simulink library "base_lib"  (R2023a)
settings: Solver=VariableStepAuto  StartTime=0.0  StopTime=10.0  RelTol=1e-3
(part 1 of 4)
settings Model: Creator=maxjo65  LastModifiedBy=maxjo65
settings SolverCC: AlgebraicLoopSolver=TrustRegion
settings OptimizationCC: ReuseModelBlockBuffer=off
settings DebuggingCC: UnconnectedInputMsg=warning  UnconnectedOutputMsg=warning  UnconnectedLineMsg=warning
settings ModelReferenceCC: EnableRefExpFcnMdlSchedulingChecks=on
settings RTWCC: DLArmComputeVersion=19.05

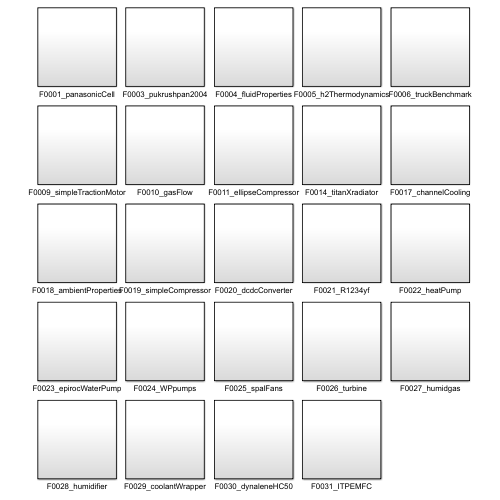
[thumbnail: Simulink's stored preview of the top-level diagram]
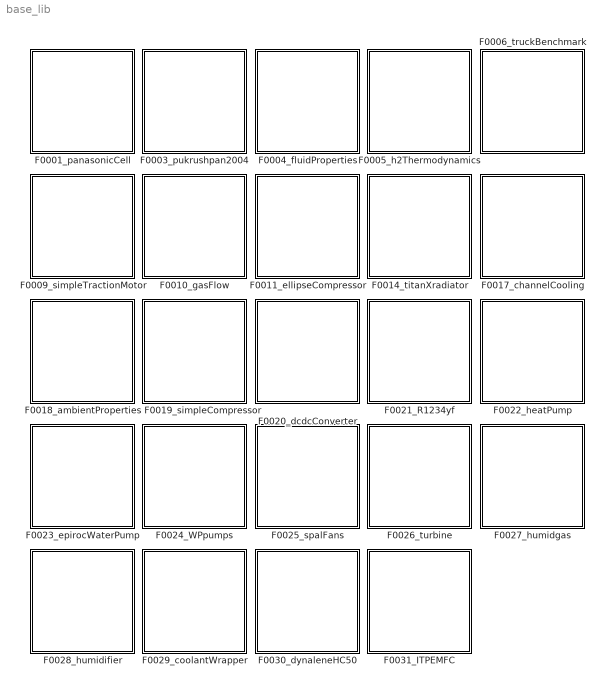
== system base_lib ==
  F0001_panasonicCell : Subsystem
  F0003_pukrushpan2004 : Subsystem
  F0004_fluidProperties : Subsystem
  F0005_h2Thermodynamics : Subsystem
  F0006_truckBenchmark : Subsystem
  F0009_simpleTractionMotor : Subsystem
  F0010_gasFlow : Subsystem
  F0011_ellipseCompressor : Subsystem
  F0014_titanXradiator : Subsystem
  F0017_channelCooling : Subsystem
  F0018_ambientProperties : Subsystem
  F0019_simpleCompressor : Subsystem
  F0020_dcdcConverter : Subsystem
  F0021_R1234yf : Subsystem
  F0022_heatPump : Subsystem
  F0023_epirocWaterPump : Subsystem
  F0024_WPpumps : Subsystem
  F0025_spalFans : Subsystem
  F0026_turbine : Subsystem
  F0027_humidgas : Subsystem
  F0028_humidifier : Subsystem
  F0029_coolantWrapper : Subsystem
  F0030_dynaleneHC50 : Subsystem
  F0031_ITPEMFC : Subsystem

== system base_lib/F0001_panasonicCell ==
  F0001_cellCapacity.m : MATLAB Function  TreatAsAtomicUnit=on
  F0001_dynamicVoltage.m : MATLAB Function  TreatAsAtomicUnit=on
  F0001_ocvSOC.m : MATLAB Function  TreatAsAtomicUnit=on

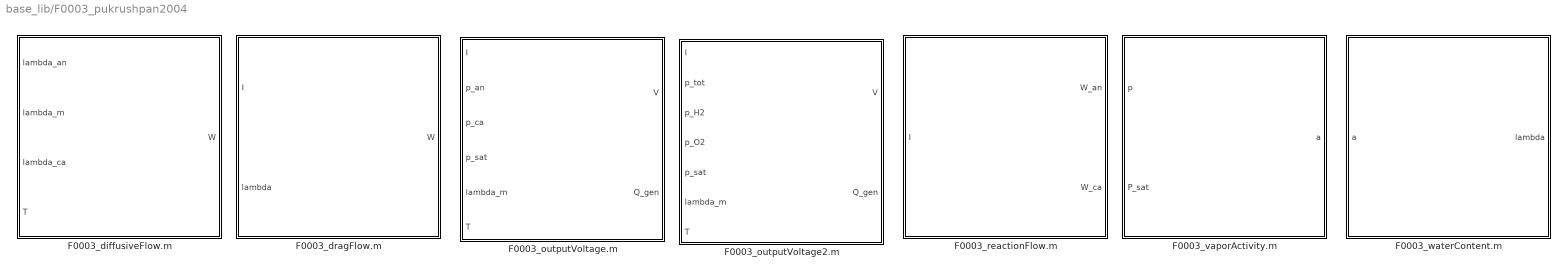
== system base_lib/F0003_pukrushpan2004 ==
  F0003_diffusiveFlow.m : MATLAB Function  TreatAsAtomicUnit=on
  F0003_dragFlow.m : MATLAB Function  TreatAsAtomicUnit=on
  F0003_outputVoltage.m : MATLAB Function  TreatAsAtomicUnit=on
  F0003_outputVoltage2.m : MATLAB Function  TreatAsAtomicUnit=on
  F0003_reactionFlow.m : MATLAB Function  TreatAsAtomicUnit=on
  F0003_vaporActivity.m : MATLAB Function  TreatAsAtomicUnit=on
  F0003_waterContent.m : MATLAB Function  TreatAsAtomicUnit=on

== system base_lib/F0004_fluidProperties ==
  F0004_mixtureMassSpecificHeat.m : MATLAB Function  TreatAsAtomicUnit=on
  F0004_pressureToMass.m : MATLAB Function  TreatAsAtomicUnit=on
  F0004_temperatureToEnthalpy.m : MATLAB Function  TreatAsAtomicUnit=on
  F0004_vaporSaturationConcentration.m : MATLAB Function  TreatAsAtomicUnit=on

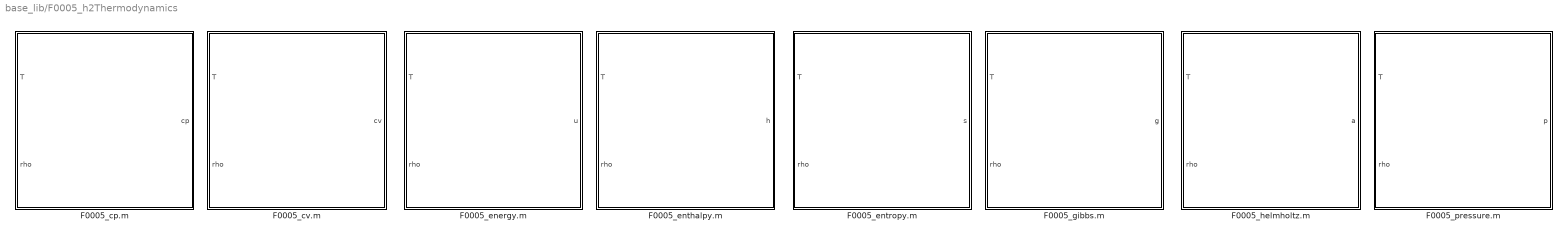
== system base_lib/F0005_h2Thermodynamics ==
  F0005_cp.m : MATLAB Function  TreatAsAtomicUnit=on
  F0005_cv.m : MATLAB Function  TreatAsAtomicUnit=on
  F0005_energy.m : MATLAB Function  TreatAsAtomicUnit=on
  F0005_enthalpy.m : MATLAB Function  TreatAsAtomicUnit=on
  F0005_entropy.m : MATLAB Function  TreatAsAtomicUnit=on
  F0005_gibbs.m : MATLAB Function  TreatAsAtomicUnit=on
  F0005_helmholtz.m : MATLAB Function  TreatAsAtomicUnit=on
  F0005_pressure.m : MATLAB Function  TreatAsAtomicUnit=on

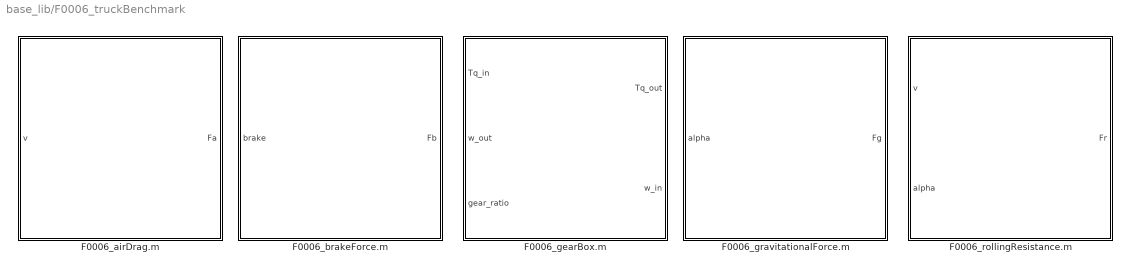
== system base_lib/F0006_truckBenchmark ==
  F0006_airDrag.m : MATLAB Function  TreatAsAtomicUnit=on
  F0006_brakeForce.m : MATLAB Function  TreatAsAtomicUnit=on
  F0006_gearBox.m : MATLAB Function  TreatAsAtomicUnit=on
  F0006_gravitationalForce.m : MATLAB Function  TreatAsAtomicUnit=on
  F0006_rollingResistance.m : MATLAB Function  TreatAsAtomicUnit=on

== system base_lib/F0009_simpleTractionMotor ==
  F0009_currentDemand.m : MATLAB Function  TreatAsAtomicUnit=on
  F0009_torque.m : MATLAB Function  TreatAsAtomicUnit=on
  F0009_torqueLimit.m : MATLAB Function  TreatAsAtomicUnit=on

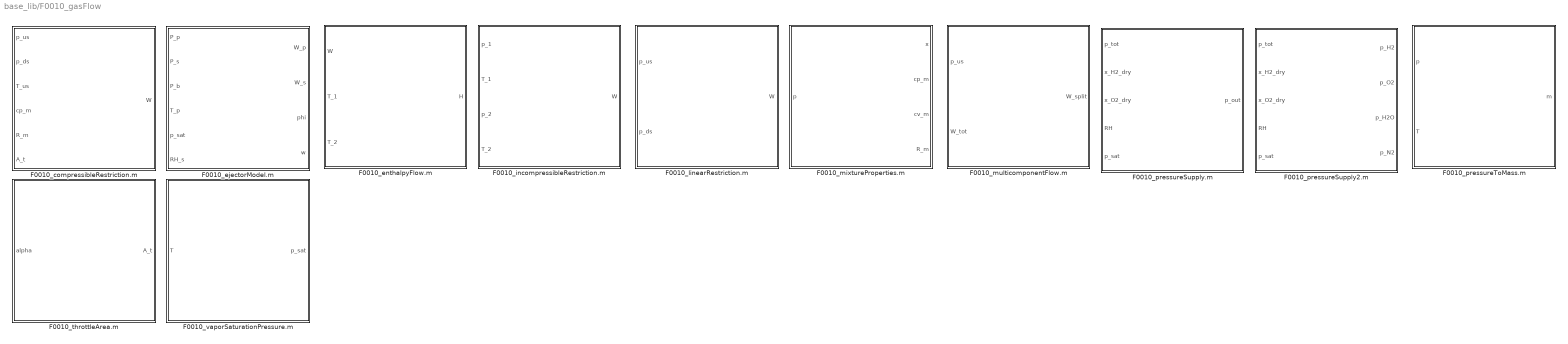
== system base_lib/F0010_gasFlow ==
  F0010_compressibleRestriction.m : MATLAB Function  TreatAsAtomicUnit=on
  F0010_ejectorModel.m : MATLAB Function  TreatAsAtomicUnit=on
  F0010_enthalpyFlow.m : MATLAB Function  TreatAsAtomicUnit=on
  F0010_incompressibleRestriction.m : MATLAB Function  TreatAsAtomicUnit=on
  F0010_linearRestriction.m : MATLAB Function  TreatAsAtomicUnit=on
  F0010_mixtureProperties.m : MATLAB Function  TreatAsAtomicUnit=on
  F0010_multicomponentFlow.m : MATLAB Function  TreatAsAtomicUnit=on
  F0010_pressureSupply.m : MATLAB Function  TreatAsAtomicUnit=on
  F0010_pressureSupply2.m : MATLAB Function  TreatAsAtomicUnit=on
  F0010_pressureToMass.m : MATLAB Function  TreatAsAtomicUnit=on
  F0010_throttleArea.m : MATLAB Function  TreatAsAtomicUnit=on
  F0010_vaporSaturationPressure.m : MATLAB Function  TreatAsAtomicUnit=on

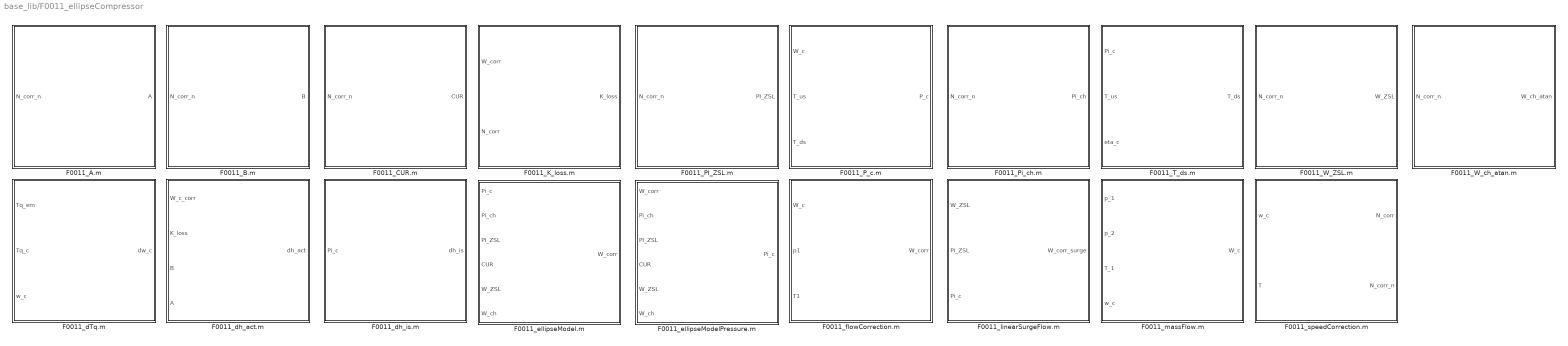
== system base_lib/F0011_ellipseCompressor ==
  F0011_A.m : MATLAB Function  TreatAsAtomicUnit=on
  F0011_B.m : MATLAB Function  TreatAsAtomicUnit=on
  F0011_CUR.m : MATLAB Function  TreatAsAtomicUnit=on
  F0011_K_loss.m : MATLAB Function  TreatAsAtomicUnit=on
  F0011_PI_ZSL.m : MATLAB Function  TreatAsAtomicUnit=on
  F0011_P_c.m : MATLAB Function  TreatAsAtomicUnit=on
  F0011_Pi_ch.m : MATLAB Function  TreatAsAtomicUnit=on
  F0011_T_ds.m : MATLAB Function  TreatAsAtomicUnit=on
  F0011_W_ZSL.m : MATLAB Function  TreatAsAtomicUnit=on
  F0011_W_ch_atan.m : MATLAB Function  TreatAsAtomicUnit=on
  F0011_dTq.m : MATLAB Function  TreatAsAtomicUnit=on
  F0011_dh_act.m : MATLAB Function  TreatAsAtomicUnit=on
  F0011_dh_is.m : MATLAB Function  TreatAsAtomicUnit=on
  F0011_ellipseModel.m : MATLAB Function  TreatAsAtomicUnit=on
  F0011_ellipseModelPressure.m : MATLAB Function  TreatAsAtomicUnit=on
  F0011_flowCorrection.m : MATLAB Function  TreatAsAtomicUnit=on
  F0011_linearSurgeFlow.m : MATLAB Function  TreatAsAtomicUnit=on
  F0011_massFlow.m : MATLAB Function  TreatAsAtomicUnit=on
  F0011_speedCorrection.m : MATLAB Function  TreatAsAtomicUnit=on

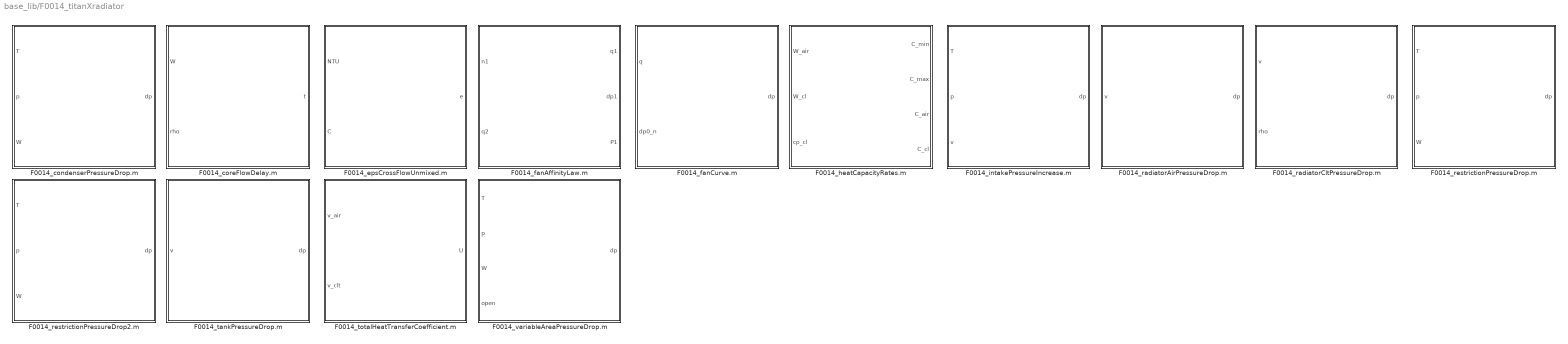
== system base_lib/F0014_titanXradiator ==
  F0014_condenserPressureDrop.m : MATLAB Function  TreatAsAtomicUnit=on
  F0014_coreFlowDelay.m : MATLAB Function  TreatAsAtomicUnit=on
  F0014_epsCrossFlowUnmixed.m : MATLAB Function  TreatAsAtomicUnit=on
  F0014_fanAffinityLaw.m : MATLAB Function  TreatAsAtomicUnit=on
  F0014_fanCurve.m : MATLAB Function  TreatAsAtomicUnit=on
  F0014_heatCapacityRates.m : MATLAB Function  TreatAsAtomicUnit=on
  F0014_intakePressureIncrease.m : MATLAB Function  TreatAsAtomicUnit=on
  F0014_radiatorAirPressureDrop.m : MATLAB Function  TreatAsAtomicUnit=on
  F0014_radiatorCltPressureDrop.m : MATLAB Function  TreatAsAtomicUnit=on
  F0014_restrictionPressureDrop.m : MATLAB Function  TreatAsAtomicUnit=on
  F0014_restrictionPressureDrop2.m : MATLAB Function  TreatAsAtomicUnit=on
  F0014_tankPressureDrop.m : MATLAB Function  TreatAsAtomicUnit=on
  F0014_totalHeatTransferCoefficient.m : MATLAB Function  TreatAsAtomicUnit=on
  F0014_variableAreaPressureDrop.m : MATLAB Function  TreatAsAtomicUnit=on

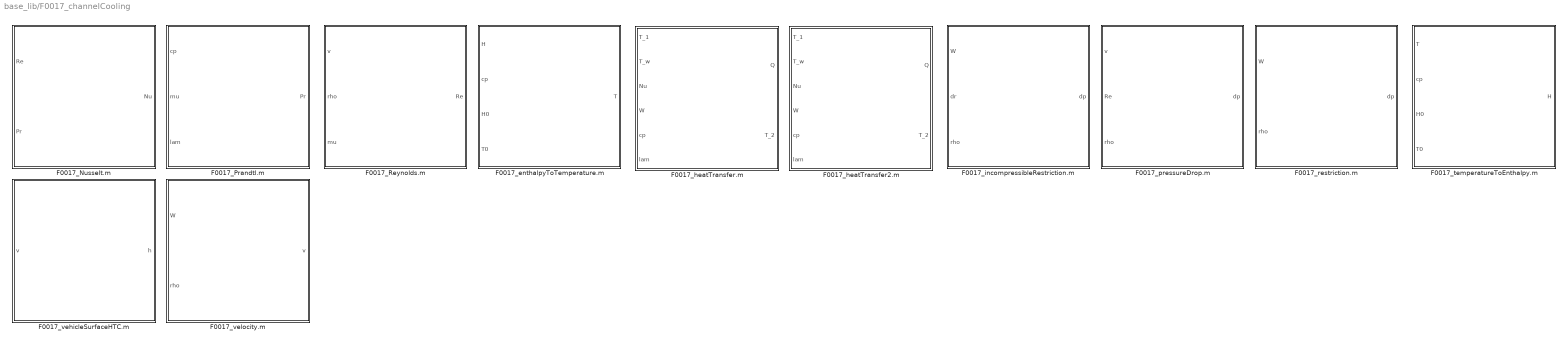
== system base_lib/F0017_channelCooling ==
  F0017_Nusselt.m : MATLAB Function  TreatAsAtomicUnit=on
  F0017_Prandtl.m : MATLAB Function  TreatAsAtomicUnit=on
  F0017_Reynolds.m : MATLAB Function  TreatAsAtomicUnit=on
  F0017_enthalpyToTemperature.m : MATLAB Function  TreatAsAtomicUnit=on
  F0017_heatTransfer.m : MATLAB Function  TreatAsAtomicUnit=on
  F0017_heatTransfer2.m : MATLAB Function  TreatAsAtomicUnit=on
  F0017_incompressibleRestriction.m : MATLAB Function  TreatAsAtomicUnit=on
  F0017_pressureDrop.m : MATLAB Function  TreatAsAtomicUnit=on
  F0017_restriction.m : MATLAB Function  TreatAsAtomicUnit=on
  F0017_temperatureToEnthalpy.m : MATLAB Function  TreatAsAtomicUnit=on
  F0017_vehicleSurfaceHTC.m : MATLAB Function  TreatAsAtomicUnit=on
  F0017_velocity.m : MATLAB Function  TreatAsAtomicUnit=on

== system base_lib/F0018_ambientProperties ==
  F0018_troposphereModel.m : MATLAB Function  TreatAsAtomicUnit=on

== system base_lib/F0019_simpleCompressor ==
  F0007_compressorPower.m : MATLAB Function  TreatAsAtomicUnit=on
  F0007_compressorTemperature.m : MATLAB Function  TreatAsAtomicUnit=on

== system base_lib/F0020_dcdcConverter ==
  F0020_dcdcConverter.m : MATLAB Function  TreatAsAtomicUnit=on

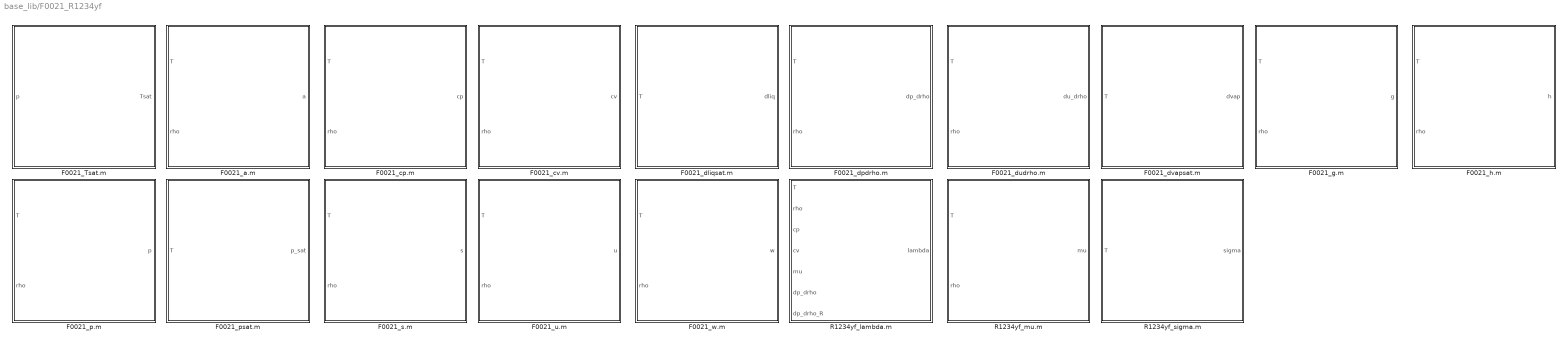
== system base_lib/F0021_R1234yf ==
  F0021_Tsat.m : MATLAB Function  TreatAsAtomicUnit=on
  F0021_a.m : MATLAB Function  TreatAsAtomicUnit=on
  F0021_cp.m : MATLAB Function  TreatAsAtomicUnit=on
  F0021_cv.m : MATLAB Function  TreatAsAtomicUnit=on
  F0021_dliqsat.m : MATLAB Function  TreatAsAtomicUnit=on
  F0021_dpdrho.m : MATLAB Function  TreatAsAtomicUnit=on
  F0021_dudrho.m : MATLAB Function  TreatAsAtomicUnit=on
  F0021_dvapsat.m : MATLAB Function  TreatAsAtomicUnit=on
  F0021_g.m : MATLAB Function  TreatAsAtomicUnit=on
  F0021_h.m : MATLAB Function  TreatAsAtomicUnit=on
  F0021_p.m : MATLAB Function  TreatAsAtomicUnit=on
  F0021_psat.m : MATLAB Function  TreatAsAtomicUnit=on
  F0021_s.m : MATLAB Function  TreatAsAtomicUnit=on
  F0021_u.m : MATLAB Function  TreatAsAtomicUnit=on
  F0021_w.m : MATLAB Function  TreatAsAtomicUnit=on
  R1234yf_lambda.m : MATLAB Function  TreatAsAtomicUnit=on
  R1234yf_mu.m : MATLAB Function  TreatAsAtomicUnit=on
  R1234yf_sigma.m : MATLAB Function  TreatAsAtomicUnit=on

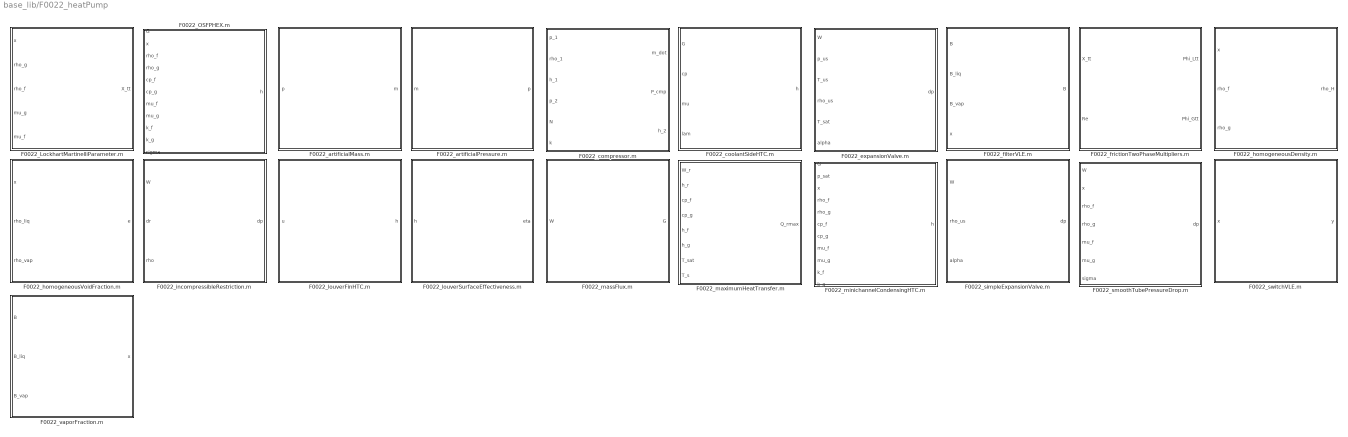
== system base_lib/F0022_heatPump ==
  F0022_LockhartMartinelliParameter.m : MATLAB Function  TreatAsAtomicUnit=on
  F0022_OSFPHEX.m : MATLAB Function  TreatAsAtomicUnit=on
  F0022_artificialMass.m : MATLAB Function  TreatAsAtomicUnit=on
  F0022_artificialPressure.m : MATLAB Function  TreatAsAtomicUnit=on
  F0022_compressor.m : MATLAB Function  TreatAsAtomicUnit=on
  F0022_coolantSideHTC.m : MATLAB Function  TreatAsAtomicUnit=on
  F0022_expansionValve.m : MATLAB Function  TreatAsAtomicUnit=on
  F0022_filterVLE.m : MATLAB Function  TreatAsAtomicUnit=on
  F0022_frictionTwoPhaseMultipliers.m : MATLAB Function  TreatAsAtomicUnit=on
  F0022_homogeneousDensity.m : MATLAB Function  TreatAsAtomicUnit=on
  F0022_homogeneousVoidFraction.m : MATLAB Function  TreatAsAtomicUnit=on
  F0022_incompressibleRestriction.m : MATLAB Function  TreatAsAtomicUnit=on
  F0022_louverFinHTC.m : MATLAB Function  TreatAsAtomicUnit=on
  F0022_louverSurfaceEffectiveness.m : MATLAB Function  TreatAsAtomicUnit=on
  F0022_massFlux.m : MATLAB Function  TreatAsAtomicUnit=on
  F0022_maximumHeatTransfer.m : MATLAB Function  TreatAsAtomicUnit=on
  F0022_minichannelCondensingHTC.m : MATLAB Function  TreatAsAtomicUnit=on
  F0022_simpleExpansionValve.m : MATLAB Function  TreatAsAtomicUnit=on
  F0022_smoothTubePressureDrop.m : MATLAB Function  TreatAsAtomicUnit=on
  F0022_switchVLE.m : MATLAB Function  TreatAsAtomicUnit=on
  F0022_vaporFraction.m : MATLAB Function  TreatAsAtomicUnit=on

== system base_lib/F0023_epirocWaterPump ==
  F0023_current.m : MATLAB Function  TreatAsAtomicUnit=on
  F0023_pressure.m : MATLAB Function  TreatAsAtomicUnit=on
  F0023_speed.m : MATLAB Function  TreatAsAtomicUnit=on

== system base_lib/F0024_WPpumps ==
  F0024_powerWP120.m : MATLAB Function  TreatAsAtomicUnit=on
  F0024_powerWP150.m : MATLAB Function  TreatAsAtomicUnit=on
  F0024_pressureWP120.m : MATLAB Function  TreatAsAtomicUnit=on
  F0024_pressureWP150.m : MATLAB Function  TreatAsAtomicUnit=on

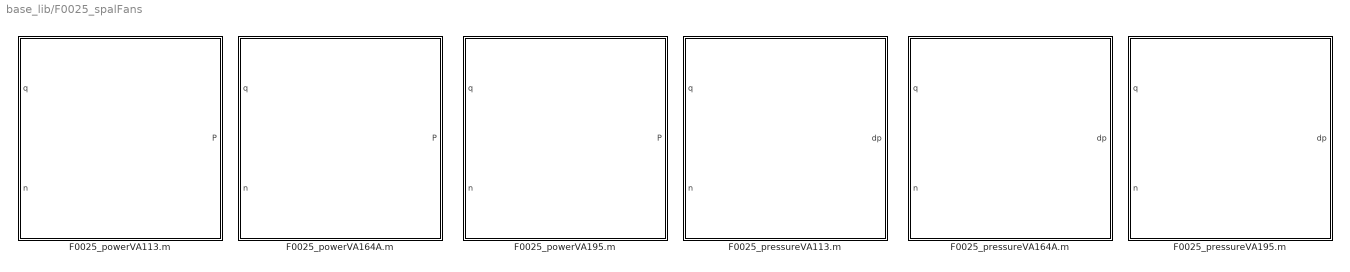
== system base_lib/F0025_spalFans ==
  F0025_powerVA113.m : MATLAB Function  TreatAsAtomicUnit=on
  F0025_powerVA164A.m : MATLAB Function  TreatAsAtomicUnit=on
  F0025_powerVA195.m : MATLAB Function  TreatAsAtomicUnit=on
  F0025_pressureVA113.m : MATLAB Function  TreatAsAtomicUnit=on
  F0025_pressureVA164A.m : MATLAB Function  TreatAsAtomicUnit=on
  F0025_pressureVA195.m : MATLAB Function  TreatAsAtomicUnit=on

== system base_lib/F0026_turbine ==
  F0026_turbine.m : MATLAB Function  TreatAsAtomicUnit=on

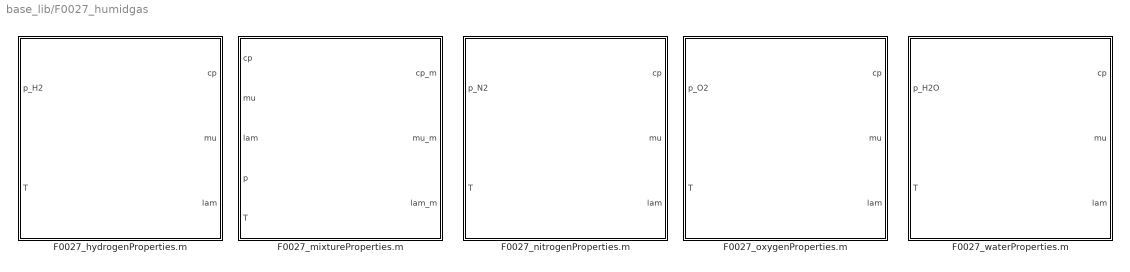
== system base_lib/F0027_humidgas ==
  F0027_hydrogenProperties.m : MATLAB Function  TreatAsAtomicUnit=on
  F0027_mixtureProperties.m : MATLAB Function  TreatAsAtomicUnit=on
  F0027_nitrogenProperties.m : MATLAB Function  TreatAsAtomicUnit=on
  F0027_oxygenProperties.m : MATLAB Function  TreatAsAtomicUnit=on
  F0027_waterProperties.m : MATLAB Function  TreatAsAtomicUnit=on

== system base_lib/F0028_humidifier ==
  F0028_absHumidity.m : MATLAB Function  TreatAsAtomicUnit=on
  F0028_heatTransfer.m : MATLAB Function  TreatAsAtomicUnit=on
  F0028_massTransfer.m : MATLAB Function  TreatAsAtomicUnit=on
  F0028_minWcp.m : MATLAB Function  TreatAsAtomicUnit=on

== system base_lib/F0029_coolantWrapper ==
  F0029_density.m : MATLAB Function  TreatAsAtomicUnit=on
  F0029_heatCapacity.m : MATLAB Function  TreatAsAtomicUnit=on
  F0029_thermalConductivity.m : MATLAB Function  TreatAsAtomicUnit=on
  F0029_viscosity.m : MATLAB Function  TreatAsAtomicUnit=on

== system base_lib/F0030_dynaleneHC50 ==
  F0030_density.m : MATLAB Function  TreatAsAtomicUnit=on
  F0030_heatCapacity.m : MATLAB Function  TreatAsAtomicUnit=on
  F0030_thermalConductivity.m : MATLAB Function  TreatAsAtomicUnit=on
  F0030_viscosity.m : MATLAB Function  TreatAsAtomicUnit=on

== system base_lib/F0031_ITPEMFC ==
  F0031_ITPEMFC.m : MATLAB Function  TreatAsAtomicUnit=on

== matlab function base_lib/F0022_heatPump/F0022_filterVLE.m ==
  data: B input; B output; B_liq input; B_vap input; x input
function B = F0022_filterVLE(B, B_liq, B_vap, x)

% assign saturated property
B( x > 0 & x < 1) = x .* B_vap + (1-x) .* B_liq;


end

== matlab function base_lib/F0022_heatPump/F0022_frictionTwoPhaseMultipliers.m ==
  data: X_tt input; Phi_Ltt output; Re input; Phi_Gtt output
function [Phi_Ltt, Phi_Gtt] = F0022_frictionTwoPhaseMultipliers(X_tt, Re)


% Liquid
Phi_Ltt = 1 + C./X_tt + 1./X_tt.^2;

% Gas
Phi_Gtt = 1 + C.*X_tt + X_tt.^2;



end

== matlab function base_lib/F0022_heatPump/F0022_homogeneousDensity.m ==
  data: x input; rho_H output; rho_f input; rho_g input
function rho_H = F0022_homogeneousDensity(x, rho_f, rho_g)

% thermopedia.com /cn/content/37/
rho_h = rho_f .* rho_g ./ ( x.* rho_f + (1-x) .* rho_g );

end

== matlab function base_lib/F0022_heatPump/F0022_homogeneousVoidFraction.m ==
  data: x input; e output; rho_liq input; rho_vap input
function e = F0022_homogeneousVoidFraction(x, rho_liq, rho_vap)

% from Engineering Data Book II, Wolverine Tube Inc.

e = 1 ./ ( 1 + (1-x)./x .* rho_vap ./ rho_liq );


end

== matlab function base_lib/F0022_heatPump/F0022_incompressibleRestriction.m ==
  data: W input; dp output; dr input; rho input; par parameter
function dp = F0022_incompressibleRestriction(W, dr, rho, par)

% parameters
C_d = par.C_d;
d   = par.d;

% restriction area
Ar = dr.^2 * pi / 4;

% diameter ratio
beta = dr./d;

% volumetric flow
Q = W ./ rho;

% pressure drop
dp = 1/2 .* rho .* (1 - beta.^4) .* (Q ./ (C_d .* Ar)).^2;

== matlab function base_lib/F0021_R1234yf/F0021_w.m ==
  data: T input; w output; rho input
function w = F0021_w(T,rho)
%R1234yf_w
%    W = R1234yf_w(T,RHO)

%    This function was generated by the Symbolic Math Toolbox version 9.3.
%    16-Oct-2023 15:47:53

t2 = T.^2;
t3 = rho.^2;
t4 = rho.^3;
t6 = rho.^5;
t8 = rho.^7;
t9 = 1.0./T;
t12 = rho./4.17e+3;
t17 = rho.*7.769784172661871e-3;
t25 = rho.*4.892086330935252e-4;
t30 = rho.*2.800959232613909e-3;
t32 = rho.*6.407673860911271e-4;
t33 = rho.*5.059952038369305e-4;
t5 = t3.^2;
t7 = t3.^3;
t10 = 1.0./t2;
t11 = t9.^3;
t13 = t9.*7.18e+2;
t14 = t9.*8.77e+2;
t15 = t9.*1.755e+3;
t16 = t9.*4.465e+3;
t18 = -t12;
t23 = t9.*5.8856e+4;
t31 = t9.*3.6785e+2;
t34 = t9.*7.94556e+4;
t35 = t3./1.73889e+7;
t40 = t9.*1.044694e+3;
t41 = t12-4.1e+1./2.5e+1;
t49 = t9.*6.54773e+2;
t50 = t9.*1.699467e+3;
t51 = t12-9.1e+1./1.0e+2;
t52 = t12-8.9e+1./1.25e+2;
t53 = t12-3.59e+2./5.0e+2;
t68 = t12-6.77e+2./1.0e+3;
t69 = t17-5.3136e+1;
t78 = t25-1.45248;
t87 = t30-8.38624;
t92 = t32-2.43152;
t100 = t33-1.42847;
t123 = t4.*t9.*9.319180196722149e-10;
t19 = -t13;
t20 = -t14;
t21 = -t15;
t22 = -t16;
t24 = exp(t18);
t42 = -t35;
t43 = t31.^(3.0./2.0);
t44 = t31.^(2.0./5.0);
t45 = t31.^(5.0./2.0);
t46 = t31.^(7.0./2.0);
t47 = t31.^(7.0./5.0);
t54 = t31-6.0./5.0;
t55 = t31.^(1.0./2.0e+1);
t56 = t41.^2;
t57 = t31.^(8.0./2.5e+1);
t59 = t31.^(1.9e+1./2.5e+1);
t61 = t31.^(3.6e+1./2.5e+1);
t62 = t31.^(1.9e+1./5.0e+1);
t63 = t31.^(4.4e+1./2.5e+1);
t65 = t31.^(6.1e+1./2.5e+1);
t66 = t31.^(4.7e+1./5.0e+1);
t67 = t23-2.048e+2;
t70 = t31-3.2e+1./2.5e+1;
t71 = t31-2.3e+1./5.0e+1;
t72 = 1.0./t31.^(3.0./1.0e+2);
t73 = t51.^2;
t74 = t52.^2;
t75 = t53.^2;
t77 = t31.^(9.7e+1./1.0e+2);
t79 = t31-6.7e+1./1.0e+2;
t80 = t31-1.13e+2./1.0e+2;
t81 = t34-2.592e+2;
t82 = t68.^2;
t85 = t31.^(9.29e+2./1.0e+3);
t97 = t40-3.2092;
t103 = t49-8.188e-1;
t106 = t50-3.0954;
t26 = exp(t19);
t27 = exp(t20);
t28 = exp(t21);
t29 = exp(t22);
t48 = exp(t42);
t58 = t55.^21;
t60 = t57.^4;
t64 = t59.^3;
t76 = t54.^2;
t83 = t70.^2;
t84 = t71.^2;
t88 = t79.^2;
t89 = t80.^2;
t90 = t56.*(8.1e+1./5.0);
t95 = t74.*(5.1e+1./5.0e+1);
t99 = t75.*(1.46e+2./2.5e+1);
t101 = t73.*(1.67e+2./1.25e+2);
t107 = t82.*(2.11e+2./2.0e+2);
t115 = t57.*1.546958;
t119 = t85.*2.355237;
t120 = rho.*t66.*2.315508393285372e-4;
t130 = t3.*t62.*3.033007263254145e-8;
t133 = rho.*t24.*t77.*3.263914628297362e-4;
t136 = t3.*t24.*t77.*3.913566700596357e-8;
t36 = t26-1.0;
t37 = t27-1.0;
t38 = t28-1.0;
t39 = t29-1.0;
t86 = t76.*1.08e+2;
t93 = -t90;
t94 = t83.*8.0e+1;
t98 = -t95;
t102 = -t99;
t104 = -t101;
t105 = t84.*(8.9e+1./1.0e+2);
t109 = t89.*(7.1e+1./5.0e+1);
t110 = -t107;
t112 = t88.*(2.31e+2./1.0e+2);
t121 = -t119;
t122 = -t120;
t131 = t48.*t64.*1.210006;
t134 = rho.*t48.*t65.*3.342232613908873e-4;
t137 = t3.*t48.*t64.*1.391699302428561e-7;
t138 = -t136;
t139 = t3.*t48.*t63.*1.06569432224005e-7;
t141 = t4.*t48.*t65.*1.922049476337705e-11;
t142 = t5.*t48.*t63.*4.085726420264459e-15;
t143 = t7.*t24.*t58.*3.588938332192827e-23;
t145 = t8.*t24.*t58.*1.229509534838242e-27;
t91 = -t86;
t96 = -t94;
t108 = -t105;
t111 = -t109;
t113 = -t112;
t132 = -t131;
t135 = -t134;
t140 = -t139;
t144 = -t143;
t114 = t91+t93;
t117 = t96+t102;
t124 = t98+t111;
t126 = t104+t113;
t127 = t108+t110;
t116 = exp(t114);
t118 = exp(t117);
t125 = exp(t124);
t128 = exp(t126);
t129 = exp(t127);
t146 = t3.*t9.*t118.*7.283294189396684e-5;
t148 = rho.*t46.*t116.*1.644384172661871e-7;
t149 = t47.*t125.*1.389966;
t150 = t11.*t128.*2.377824987227386e+7;
t152 = t3.*t46.*t129.*3.407663509480186e-8;
t154 = t4.*t9.*t87.*t118.*5.821977769301905e-9;
t155 = t3.*t46.*t69.*t116.*1.971683660266032e-11;
t157 = rho.*t47.*t78.*t125.*3.333251798561151e-4;
t159 = rho.*t11.*t92.*t128.*5.702218194789895e+3;
t160 = t4.*t46.*t100.*t129.*2.723951646267135e-12;
t147 = -t146;
t151 = -t150;
t153 = -t152;
t156 = -t155;
t158 = -t157;
t161 = t115+t121+t122+t123+t130+t132+t133+t135+t137+t138+t140+t141+t142+t144+t145+t147+t148+t149+t151+t153+t154+t156+t158+t159+t160;
et1 = t66.*9.65567e-1+t138+t145-rho.*t62.*2.529528057553957e-4-t3.*t9.*1.165829442609941e-5-t24.*t77.*1.3610524;
et2 = t48.*t65.*1.393711-t46.*t116.*6.857082e-4+t87.*t154+t92.*t159+t100.*t160+rho.*t24.*t77.*6.527829256594724e-4+rho.*t48.*t63.*8.887890647482015e-4;
et3 = rho.*t48.*t64.*(-1.741015827338129e-3)+rho.*t9.*t118.*6.074267353956834e-1-rho.*t11.*t128.*1.52363270164786e+4+rho.*t47.*t125.*6.799833669064748e-4;
et4 = rho.*t46.*t129.*2.841991366906475e-4+t6.*t24.*t58.*8.979523707146454e-19-t7.*t24.*t58.*7.177876664385654e-23;
et5 = t4.*t48.*t63.*(-1.192623542075196e-10)-t3.*t48.*t65.*4.007473158164116e-7+t4.*t48.*t64.*6.674816798218516e-11+t6.*t48.*t63.*1.95958101691341e-18;
et6 = t5.*t48.*t65.*9.218462716247988e-15-t4.*t9.*t118.*6.800070034544626e-8+t3.*t46.*t116.*6.388255059261943e-10;
et7 = t4.*t46.*t129.*(-5.747537973623655e-12)-t11.*t92.*t128.*4.755649974454772e+7+t47.*t78.*t125.*2.779932+rho.*t46.*t69.*t116.*3.288768345323741e-7;
et8 = t3.*t9.*t87.*t118.*(-1.456658837879337e-4)-t3.*t46.*t100.*t129.*6.815327018960372e-8-rho.*t47.*t78.^2.*t125.*3.333251798561151e-4-t3.*t46.*t69.^2.*t116.*1.971683660266032e-11;
et9 = t4.*2.533418566459739e-12-t48.*t60.*2.75881368-t3.*t118.*1.979963079895795e-7-t10.*t128.*1.93923473200548e+5;
et10 = t44.*t125.*1.9459524+t67.*t146+t81.*t155+t97.*t157+t103.*t152+t106.*t150-rho.*t72.^2.*2.176577889688249e-4+t3.*1.0./t31.^(3.1e+1./5.0e+1).*1.152542760036575e-8+1.0./t31.^(1.7e+1./2.5e+1).*4.9502656e-1;
et11 = 1.0./t31.^(7.1e+1./1.0e+3).*(-2.188015173)+rho.*t24.*t72.*3.165997189448441e-4-rho.*t48.*t61.*8.155047577937649e-4+rho.*t45.*t116.*5.755344604316547e-7;
et12 = t7.*t24.*t55.*(-3.768385248802469e-23)+t8.*t24.*t55.*1.290985011580154e-27-t3.*t24.*t72.*3.796159699578467e-8;
et13 = t3.*t48.*t59.*(-1.875622007142488e-7)+t3.*t48.*t60.*3.173074409537118e-7+t5.*t48.*t59.*7.190878499665448e-15+t4.*t48.*t61.*4.689800722264001e-11;
et14 = t3.*t45.*t129.*(-1.192682228318065e-7)+t4.*t87.*t118.*1.582704300476255e-11-t47.*t97.*t125.*1.389966+rho.*t10.*t92.*t128.*4.650443002411223e+1;
et15 = rho.*t46.*t81.*t116.*(-1.644384172661871e-7)-rho.*t44.*t78.*t125.*4.666552517985612e-4-t3.*t45.*t69.*t116.*6.900892810931111e-11+t4.*t45.*t100.*t129.*9.533830761934972e-12;
et16 = rho.*t11.*t92.*t106.*t128.*(-5.702218194789895e+3)-t4.*t9.*t67.*t87.*t118.*5.821977769301905e-9-t4.*t46.*t100.*t103.*t129.*2.723951646267135e-12;
et17 = t2.*3.653734124219459e-5+1.0./t36.^2.*exp(t9.*-1.436e+3).*2.876052391546904e+1+1.0./t37.^2.*exp(t9.*-1.754e+3).*8.736380352244283+1.0./t38.^2.*exp(t9.*-3.51e+3).*1.696916093943165e+2+1.0./t39.^2.*exp(t9.*-8.93e+3).*2.990869359808914e+2+rho.*t72.^56.*8.072375558752998e-5;
et18 = rho.*1.0./t31.^1.071.*(-3.72539753676259e-5)-(t26.*2.876052391546904e+1)./t36-(t27.*8.736380352244283)./t37-(t28.*1.696916093943165e+2)./t38-(t29.*2.990869359808914e+2)./t39;
et19 = t4.*t72.^54.*5.712042455816759e-13-t3.*1.0./t31.^(5.3e+1./5.0e+1).*1.565883373876438e-9+rho.*t31.^(7.0./2.5e+1).*t48.*8.468300984172661e-4;
et20 = rho.*1.0./t55.^12.*t125.*(-1.866621007194245e-4)+t8.*t24.*1.0./t55.^19.*6.454925057900768e-29+t3.*t31.^(1.1e+1./2.5e+1).*t48.*1.408065768852544e-7;
et21 = t4.*t48.*t72.^8.*1.139466607056987e-11+t3.*t24.*1.0./t31.^(1.03e+2./1.0e+2).*1.13884790987354e-9+rho.*t9.*t128.*2.528445291510791e-1;
et22 = rho.*t11.*t128.*(-2.634424805992931e+4)+rho.*t47.*t125.*9.466435107913669e-4-t4.*t9.*t118.*9.315164430883049e-7;
et23 = t3.*t43.*t116.*(-1.725223202732778e-10)+t3.*t46.*t116.*4.258836706174629e-9+t4.*t43.*t129.*2.383457690483743e-11-t4.*t46.*t129.*4.8486339303555e-12;
et24 = t4.*t67.*t118.*(-3.165408600952511e-11)-rho.*t10.*t106.*t128.*9.300886004822446e+1+rho.*t44.*t97.*t125.*9.333105035971223e-4+t3.*t45.*t81.*t116.*1.380178562186222e-10;
et25 = t4.*t45.*t103.*t129.*(-1.906766152386994e-11)+rho.*t11.*t106.^2.*t128.*5.702218194789895e+3-rho.*t47.*t97.^2.*t125.*3.333251798561151e-4;
et26 = t4.*t9.*t67.^2.*t118.*5.821977769301905e-9-t3.*t46.*t81.^2.*t116.*1.971683660266032e-11+t4.*t46.*t103.^2.*t129.*2.723951646267135e-12;
w = sqrt(T.*((rho.*t161)./2.085e+3-(t3.*(et1+et2+et3+et4+et5+et6+et7+et8))./1.73889e+7+(t2.*(t12.*t161-rho.*t9.*(et9+et10+et11+et12+et13+et14+et15+et16).*8.821342925659472e-2+1.0).^2.*7.39023892439211e-6)./(et17+et18+et19+et20+et21+et22+et23+et24+et25+et26)+1.0).*7.290736472421491e+1);
end

== matlab function base_lib/F0004_fluidProperties/F0004_mixtureMassSpecificHeat.m ==
  data: p input; cp output; cv output; par parameter
function [cp, cv] = F0004_mixtureMassSpecificHeat(p, par)
% total pressure
p_tot = sum(p);

% mass specific heat capacity
cp_r  = par.cp_r;
cp_v  = par.cp_H2O;
cp_N2 = par.cp_N2;
R_r    = par.R_r;
R_H2O  = par.R_H2O;
R_N2   = par.R_N2;

% partial pressures
p_r  = p(1);
p_v  = p(2);
p_N2 = p(3);

% mole fractions
x_r   = p_r  ./ p_tot;
x_v   = p_v  ./ p_tot;
x_N2  = p_N2 ./ p_tot;

% average mass
M_avg = sum([x_r, x_v, x_N2] .* [par.M_r, par.M_H2O, par.M_N2]);

% mole fraction to mass fraction
w_r   = x_r  .* par.M_r   ./ M_avg;
w_v   = x_v  .* par.M_H2O ./ M_avg;
w_N2  = x_N2 .* par.M_N2  ./ M_avg;

% mixture gas constant
Rm = w_r.*R_r + w_v.*R_H2O + w_N2 .* R_N2;

% ideal mixture heat capacity
cp = w_r.*cp_r + w_v.*cp_v + w_N2 .* cp_N2;
cv = cp - Rm;

end

== matlab function base_lib/F0021_R1234yf/R1234yf_lambda.m ==
  data: T input; lambda output; rho input; cp input; cv input; mu input; dp_drho input; dp_drho_R input
function lambda = R1234yf_lambda(T, rho, cp, cv, mu, dp_drho, dp_drho_R)


% Critical point & molar mass
Tc   =     367.85; % [K]
pc   = 	3382200.0; % [Pa]
rhoc =     4170.0; % [mol/m3]
M    = 0.1140415928; % [kg/mol]
% R    = 8.314472;

% change units
rhoc = rhoc .* M;
rho  = rho  .* M;

% coefficients
A = [-0.0102778; 0.0291098; 0.000860643];

B      = zeros(5,2);
B(1,1) = -0.0368219;
B(1,2) =  0.0397166;
B(2,1) =  0.0883226;
B(2,2) = -0.0772390;
B(3,1) = -0.0705909;
B(3,2) =  0.0664707;
B(4,1) =  0.0259026;
B(4,2) = -0.0249071;
B(5,1) = -0.00322950;
B(5,2) =  0.00336228;


% Dilute-gas thermal conductivity
lambda_0 = sum( repmat(A', length(T), 1) .* (T./Tc).^(0:2), 2 );

% residual thermal conductivity
lambda_r = sum( (  repmat(B(:,1)', length(T), 1) + ...
    repmat(B(:,2)', length(T), 1) .* repmat((T./Tc), 1, 5) ) .* ...
    (rho./rhoc).^(1:5), 2);

% critical enhancement
R0        = 1.03;
kb        = 1.380649e-23;
eta       = mu;
T_R       = 1.5 .* Tc;
gam       = 1.239;
nu        = 0.63;
GAM       = 0.0496;
xi0       = 1.94e-10;
qd        = 0.5835e9;
dp_drho   = dp_drho   ./ M;
dp_drho_R = dp_drho_R ./ M;
drho_dp   = 1 ./ dp_drho;
drho_dp_R = 1 ./ dp_drho_R;


xi = xi0 .* ( pc .* rho ./ (GAM .* rhoc.^2) ).^(nu./gam) .* ...
            (  max(drho_dp - (T_R./T) .* drho_dp_R,eps)  ).^(nu./gam);


omega0    = 2./pi .* (1 - exp(-1./ ( 1./(qd.*xi) + (1/3) .* (qd.*xi.*rhoc./rho).^2 ) ) );
omega     = 2./pi .* (  (cp-cv)./cp .* atan(qd.*xi) + cv./cp .* qd.*xi );
dlambda_c = rho .* cp .* R0 .* kb .* T ./ (6 .* pi .* eta .* xi) .* (omega-omega0);

lambda = lambda_0 + lambda_r + dlambda_c;

end

== matlab function base_lib/F0021_R1234yf/R1234yf_mu.m ==
  data: T input; mu output; rho input
function mu = R1234yf_mu(T,rho)

% Critical point & molar mass
Tc   =     367.85; % [K]
% pc   = 	3382200.0; % [Pa]
rhoc =     4170.0; % [mol/m3]
% M    = 0.1140415928; % [kg/mol]
% R    = 8.314472;

% Viscosity coefficients
a0 = -836950;
a1 = 6336.28;
a2 = -2.3547;
a3 = 0.0395563;
a4 = 39509.1;
a5 = 121.018;

b0 = -19.572881;
b1 = 219.73999;
b2 = -1015.3226;
b3 = 2471.0125;
b4 = -3375.1717;
b5 = 2491.6597;
b6 = -787.26086;
b7 = 14.085455;
b8 = -0.34664158;

b = [b0; b1; b2; b3; b4; b5; b6];

c0 = -0.19425910;
c1 = -2.079577245;
c2 = 0;
c3 = -43.47027288;
c4 = 0;
c5 = 0;
c6 = 0;
c7 = -3.53682791;
c8 = 1;

% dilute-gas limit viscosity
eta0 = (a0 + a1 .* T + a2 .* T.^2 + a3 .* T.^3) ./ (a4 + a5 .* T + T.^2);

% temperature dependent contribution
sigma   = 0.531e-9;
e_kb    = 275;
Mw      = 114.0416e-3;
N_a     = 6.02214076e23;
T_star  =  T ./ e_kb;
Bn_star = sum(  repmat(b', length(T), 1) .* T_star.^(-0.25.*(0:6)) , 2) + b7 .* T_star.^(-2.5) + b8 .* T_star.^-5.5; 
Bn      = Bn_star .* N_a .* sigma.^3;
eta1    = Bn .* eta0;

% residual term
rhor = rho ./ rhoc;
Tr    = T ./ Tc;

deta = rhor.^(2/3) .* Tr.^(1/2) .* ...
                (c0 + c1 .* rhor + c2 .* rhor.^2 +  ... 
                        (c3 .* rhor + c4 .* rhor.^6 + c5 .* rhor .* Tr.^2 + c6 .* rhor.^5 .* Tr) ./ (c7 .* Tr + c8 .* rhor .* Tr) );


% total viscosity
eta = eta0 + eta1 .* rho + deta;

% SI units
mu = eta .* 1e-6;

end

== matlab function base_lib/F0022_heatPump/F0022_louverFinHTC.m ==
  data: u input; h output; par parameter
function h = F0022_louverFinHTC(u, par)

% HEX Geometry
% L_a = 23;       % Louver angle [degrees]
% F_p = 1.4e-3;   % Fin pitch [m]
% L_p = 1.7e-3;   % Louver pitch [m]
% L_l = 6.4e-3;   % Louver length [m]
% H   = 8.15e-3;  % Fin height [m]
% T_p = 10.15e-3; % Tube pitch [m]
% T_d = 16e-3;    % Tube depth [m]
% d_f = 0.1e-3;   % Fin thickness [m]
% F_d = 16e-3;    % flow depth

% contraction ratio
sigma = par.sigma;

% Air properties
cp  = par.cp_air;
v   = par.v_air;
rho = par.rho_air;

% HEX Geometry parameters
L_a  = par.L_a;  % Louver angle [deg]
F_p  = par.F_p;  % Fin pitch [m]
L_p  = par.L_p;  % Louver pitch [m]
L_l  = par.L_l;  % Louver length [m]
H    = par.H;    % Fin height [m]
T_p  = par.T_p;  % Tube pitch [m]
% T_d  = par.T_d;  % Tube depth [m]
d_f  = par.d_f;  % Fin thickness [m]
F_d  = par.F_d;  % Flow depth [m]

% Prandtl number
P_r = 0.7;

% minimum air velocity
u = max(0.001, u);

% maximum air velocity
V_c = u .* sigma;

% Air side Reynolds number based on Louver pitch
Re = V_c .* L_p ./ v;

% Colburn j-factor correlation
j = Re.^(-0.487) .* (L_a./90).^(0.257) * ...
    (F_p./L_p).^(-0.13) .* (H ./ L_p).^(-0.29) .* ...
    (F_d ./ L_p).^(-0.235) .* (L_l./L_p).^(0.68) .* ...
    (T_p./L_p).^(-0.279) .* (d_f./L_p).^(-0.05);


% HTC
h = j .* rho .* V_c .* cp ./ P_r.^(2/3);

end

== matlab function base_lib/F0022_heatPump/F0022_louverSurfaceEffectiveness.m ==
  data: h input; eta output; par parameter
function eta = F0022_louverSurfaceEffectiveness(h, par)

% HEX Geometry parameters
H    = par.H;    % Fin height [m]
d_f  = par.d_f;  % Fin thickness [m]
F_d  = par.F_d;  % Flow depth [m]

% Areas
A_f = par.A_f;
A_o = par.A_o;


% aluminium properties
k = par.k_w;


% Fin efficiency
m     = sqrt( 2.*h ./ (k .* d_f) .* (1 + d_f./F_d) );
l     = H/2 - d_f;
eta_f = tanh(m*l) ./ m.*l;

% Surface effectiveness
eta   = 1 - A_f ./ A_o .* (1 - eta_f);

end

== matlab function base_lib/F0021_R1234yf/R1234yf_sigma.m ==
  data: T input; sigma output
function sigma = R1234yf_sigma(T)

% Critical point & molar mass
Tc   =     367.85; % [K]
% pc   = 	3382200.0; % [Pa]
% rhoc =     4170.0; % [mol/m3]
% M    = 0.1140415928; % [kg/mol]
% R    = 8.314472;

% max & min temperature
T = max(T,  0);
T = min(T, Tc);

% coefficients
c = [ 42.36234 0.60895 -0.42621 367.85]';

% surface tension
Tr      = T ./ Tc; 
sigma = c(1) .* (1 - Tr).^1.26 .* ( 1 + c(2).*(1-Tr).^0.5 + c(3).*(1-Tr) );

% shift to SI unit
sigma = sigma * 1e-3;

end

== matlab function base_lib/F0022_heatPump/F0022_massFlux.m ==
  data: W input; G output; par parameter
function G = F0022_massFlux(W, par)

% parameters
D_h = par.D_h;

% mass flux
G = 4 .* W ./ (D_h.^2 .* pi);
end

== matlab function base_lib/F0022_heatPump/F0022_maximumHeatTransfer.m ==
  data: W_r input; Q_rmax output; h_r input; cp_f input; cp_g input; h_f input; h_g input; T_sat input; T_s input
function Q_rmax = F0022_maximumHeatTransfer(W_r, h_r, cp_f, cp_g, h_f, h_g, T_sat, T_s)

if T_sat <= T_s
    % Evaporation
    h_fg = max(h_g - h_r, 0);
    
    % superheating
    h_sup = cp_g .* (T_s - T_sat);

    % maximum heat transfer
    Q_rmax = W_r .* (h_fg + h_sup);
else
    % Condensation
    h_fg = max(h_r - h_f, 0);

    % subcooling
    h_sub = cp_f .* (T_sat - T_s);
    
    % maximum heat transfer
    Q_rmax = W_r .* (h_fg + h_sub);
end

== matlab function base_lib/F0022_heatPump/F0022_minichannelCondensingHTC.m ==
  data: G input; h output; p_sat input; x input; rho_f input; rho_g input; cp_f input; cp_g input; mu_f input; mu_g input; k_f input; k_g input; par parameter
function h = F0022_minichannelCondensingHTC(G, p_sat,  x, rho_f, rho_g, cp_f, cp_g, mu_f, mu_g, k_f, k_g, par)
% Critical point & molar mass
pc = par.pc;

% gravity
g = 9.82;

% channel dimensions
b = par.b;
a = par.a;

% hydraulic diameter
D_h =  2 .* a .* b ./ (a + b);

G = max(G,0);

% Liquid reynolds & prandtl numbers
Re_f = (1-x) .* G .* D_h ./ mu_f;
Pr_f = cp_f .* mu_f ./ k_f;

% liquid only heat transfer coefficient
h_f = 0.023 .* Re_f.^0.8 .* Pr_f.^0.4 .* k_f ./ D_h;

% Gas only reynolds & prandtl numbers
Re_g = x .* G .* D_h ./ mu_g;
Pr_g = cp_g .* mu_g ./ k_g;



% gas only heat transfer coefficient
h_g = 0.023 .* Re_g.^0.8 .* Pr_g.^0.4 .* k_g ./ D_h;

% reduced pressure
p_r = p_sat ./ pc;

% Shah correlating parameter
% Z = (1./max(min(x,1),0.0000001) - 1).^0.8 .* p_r.^0.4;

Z = ( (1-x)./(x+0.00001) ).^0.8 .* p_r.^0.4;

% Regime depenedent HTCs
h_I = h_f .* (1 + 3.8./(Z.^0.95 + 0.00001)) .* ...
    (mu_f ./ (14 .* mu_g)).^(0.0058 + 0.557 .* p_r);


% smooth transition to subcooled liquid & superheated vapor
y = (x+0.1) / 0.2;
y = tanh(y*2)/2 + 1/2;
z =  (x-0.8) / 0.1;
z = tanh(z*2)/2 + 1/2;

% HTC
h = h_I .* y .* (1-z) + h_f .* (1-y) + h_g .* z;


% h_nu = 1.32 .* Re_f.^(-1/3) .* ...
%     (  rho_f .* (rho_f - rho_g) .* g .* k_f.^3 ./ mu_f.^2   ).^(1/3);
% 
% % dimensionless vapor velocity
% J_g = x.*G ./ (g.*D_h.*rho_g.*(rho_f - rho_g)).^0.5;
% 
% % Single phase regimes
% SP_REG1 = x == 0;
% SP_REG2 = x == 1;
% TP_REG1 = (~SP_REG1) & (~SP_REG2);
% 
% % % Two-phase regimes
% % TP      =  (x>0) & (x<1); 
% 
% % % vertical flow
% % TP_REG1 = TP & (J_g >= 1./(2.4.*Z + 0.73));
% % TP_REG3 = TP & (J_g <= 0.89 - 0.93 .* exp(-0.987 .* Z.^(-1.17)));
% % TP_REG2 = TP & (~TP_REG1 & ~TP_REG3);
% 
% % % horizontal flow
% % TP_REG1 = TP & (J_g >= 0.98 .* (Z + 0.263).^(-0.62) );
% % TP_REG3 = TP & (J_g <= 0.95 .* (1.254 + 2.27 .* Z.^1.249 ).^(-1) );
% % TP_REG2 = TP & (~TP_REG1 & ~TP_REG3);
% 
% % Output
% h = zeros(size(x));
% h( SP_REG1 ) = h_f( SP_REG1 );
% h( SP_REG2 ) = h_g( SP_REG2 );
% h( TP_REG1 ) = h_I( TP_REG1 );
% % h( TP_REG2 ) = h_I( TP_REG2 ) + h_nu( TP_REG2 );
% % h( TP_REG3 ) = h_nu( TP_REG3 );

end

== matlab function base_lib/F0022_heatPump/F0022_simpleExpansionValve.m ==
  data: W input; dp output; rho_us input; alpha input; par parameter
function dp = F0022_simpleExpansionValve(W, rho_us, alpha, par)

% parameters
M  = par.M;
Tc = par.Tc;
D  = par.D;
C  = par.C;

% constants
R = 8.314472;

% exv geometry
A = alpha .* D.^2 .* pi / 4;

% pressure drop
dp = 1./rho_us .* ( W ./ (C.*A) ).^2;

end

== matlab function base_lib/F0004_fluidProperties/F0004_pressureToMass.m ==
  data: p input; m output; T input; par parameter
function m = F0004_pressureToMass(p, T, par)
% gas constants
R_r    = par.R_r;
R_H2O  = par.R_H2O;
R_N2   = par.R_N2;
Rj     = [R_r; R_H2O; R_N2];
V      = par.V;

% mass
m = p .* V ./ (Rj .* T);
end

== matlab function base_lib/F0023_epirocWaterPump/F0023_current.m ==
  data: q input; I output; V input
function I = F0023_current(q, V)

% parameters
a = [-4.6456; 2.8036; 1.7966];

% function
I = a(1) + a(2) .* q + a(3) .* V; 

end

== matlab function base_lib/F0023_epirocWaterPump/F0023_pressure.m ==
  data: q input; dp output; V input
function dp = F0023_pressure(q, V)

% parameters
a = [-0.1990; 0.2290; 0.1984; -0.0313; -0.2935];

% function
dp = a(1) + a(2) .* q + a(3) .* V + a(4) .* q.* V + a(5) .* q.^2;

end

== matlab function base_lib/F0017_channelCooling/F0017_temperatureToEnthalpy.m ==
  data: T input; H output; cp input; H0 input; T0 input; par parameter
function H = F0017_temperatureToEnthalpy(T, cp, H0, T0, par)
   
    % enthalpy
    H = H0 + cp.*(T - T0);

end

== matlab function base_lib/F0023_epirocWaterPump/F0023_speed.m ==
  data: q input; w output; V input
function w = F0023_speed(q, V)

% parameters
b = [1.6954; 0.3962; 0.4124; -0.0700];

% function
w = 1000 * (b(1) + b(2) .* q + b(3) .* V + b(4) .* q.* V) .* 2.*pi/60; 

end

== matlab function base_lib/F0024_WPpumps/F0024_powerWP120.m ==
  data: q input; P output; n input
function P = F0024_powerWP120(q, n)

% parameters
a = [-385.2919; 155.7472; 0.1219];

% function
P = a(1) + a(2) .* q + a(3) .* n; 

end

== matlab function base_lib/F0024_WPpumps/F0024_powerWP150.m ==
  data: q input; P output; n input
function P = F0024_powerWP150(q, n)

% parameters
a =  [-1578.62293476575; 122.984201937838; 0.569192422324180];

% function
P = a(1) + a(2) .* q + a(3) .* n; 

end

== matlab function base_lib/F0024_WPpumps/F0024_pressureWP120.m ==
  data: q input; dp output; n input
function dp = F0024_pressureWP120(q, n)

% parameters
a = 1.0e+04 * [0.8098; 0.0038; 0.0013; -5.4000];

% function
dp = a(1) + a(2) .* n + a(3) .* q.* n + a(4) .* q.^2;

end

== matlab function base_lib/F0024_WPpumps/F0024_pressureWP150.m ==
  data: q input; dp output; n input
function dp = F0024_pressureWP150(q, n)

% parameters
a = [-123461.665683305;
    69.1858073291126; 3.37203190426057; -3645.86929609208];

% function
dp = a(1) + a(2) .* n + a(3) .* q.* n + a(4) .* q.^2;

end

== matlab function base_lib/F0025_spalFans/F0025_powerVA113.m ==
  data: q input; P output; n input
function P = F0025_powerVA113(q, n)

% parameters
c = [921.12; -758.93; 1081.5; -464.8];

% function
P2 = c(1) + c(2) .* q + c(3) .* q.^2 + c(4) .* q.^3;

% affinity law
P = P2 .* (n./4750).^3;

end

== matlab function base_lib/F0025_spalFans/F0025_powerVA164A.m ==
  data: q input; P output; n input
function P = F0025_powerVA164A(q, n)

% parameters
c = [1.304309138899855e+03; -1.023894573709462e+02];

% function
P2 = c(1) + c(2) .* q.^2;


% affinity law
P = P2 .* (n./3000).^3;

end

== matlab function base_lib/F0014_titanXradiator/F0014_totalHeatTransferCoefficient.m ==
  data: v_air input; U output; v_clt input; par parameter
function U = F0014_totalHeatTransferCoefficient(v_air, v_clt, par)

% parameters
cU    = par.cU;
cUexp = par.cUexp;

% saturation
v_air = max(v_air, 0);
v_clt = max(v_clt, 0);


% Heat transfer coefficient
temp = cU(1) + cU(2) .* v_air.^-cUexp(1) + cU(3)*v_clt .^ -cUexp(2);
U    = 1./temp;

== matlab function base_lib/F0004_fluidProperties/F0004_temperatureToEnthalpy.m ==
  data: T input; h output; par parameter
function h = F0004_temperatureToEnthalpy(T, par)
% output size
h = zeros(3,1);

% mass heat capacity
cp_r  = par.cp_r;
cp_v  = par.cp_H2O;
cp_N2 = par.cp_N2;
cp    = [cp_r; cp_v; cp_N2];

% specific enthalpy
h = cp .* T;
end

== matlab function base_lib/F0025_spalFans/F0025_powerVA195.m ==
  data: q input; P output; n input
function P = F0025_powerVA195(q, n)

% parameters
c = [33.581405740918410; -4.335839924811192e+02];

% function
P2 = c(1) + c(2) .* q.^2;


% affinity law
P = P2 .* (n./5000).^3;

end

== matlab function base_lib/F0025_spalFans/F0025_pressureVA113.m ==
  data: q input; dp output; n input
function dp = F0025_pressureVA113(q, n)

% parameters
a = [859.99; -171.19; -292.55];

% function
dp2 = a(1) + a(2) .* q + a(3) .* q.^2;

% affinity law
dp = dp2 .* (n./4750).^2;

end

== matlab function base_lib/F0017_channelCooling/F0017_vehicleSurfaceHTC.m ==
  data: v input; h output; par parameter
function h = F0017_vehicleSurfaceHTC(v, par)

h = 0.6 + 6.64 .* sqrt(v);

end

== matlab function base_lib/F0022_heatPump/F0022_smoothTubePressureDrop.m ==
  data: W input; dp output; x input; rho_f input; rho_g input; mu_f input; mu_g input; sigma input; par parameter
function dp = F0022_smoothTubePressureDrop(W, x, rho_f, rho_g, mu_f, mu_g, sigma, par)

% parameters
D = par.D;
L = par.L;

% gravitation
g = 9.82;

% minimum mass flux
W = max(W, 1e-4);

% mass flux
G_tp = 4.*W ./ (pi.*D.^2);

% liquid-only friction factor
Re_lo = G_tp .* D ./ mu_f;
f_lo  = 0.25 .* ( log10(  150.39 ./ (Re_lo.^0.98865) - 152.66./(Re_lo)  ) ).^(-2);

% gas-only friction factor
Re_go = G_tp .* D ./ mu_g;
f_go  = 0.25 .* ( log10(  150.39 ./ (Re_go.^0.98865) - 152.66./(Re_go)  ) ).^(-2);

% Laplace constant
La = sqrt( sigma ./ (g.*(rho_f - rho_g) ) ) ./ D;

% liquid-only pressure gradient
dp_dz_lo = G_tp.^2 ./(2.*D.*rho_f) .* f_lo;

% gas-only pressure gradient
dp_dz_go = G_tp.^2 ./(2.*D.*rho_g) .* f_go;

% two phase multiplier
Y       = sqrt(dp_dz_go ./ dp_dz_lo);
phi2_lo = (Y.^2 .* x.^3 + (1-x).^(1/3) .* (1+2.*x.*(Y.^2 -1)) ) .* ...
    (1 + 1.54 .*(1-x).^0.5 .* La.^1.47); 

% two-phase pressure gradient
dp_dz_tp = dp_dz_lo .* phi2_lo; 

% pressure drop
dp = dp_dz_tp .* L;

end

== matlab function base_lib/F0022_heatPump/F0022_switchVLE.m ==
  data: x input; y output
function y = F0022_switchVLE(x)
% step function on 0-1
y = tanh( 1000*(x-0.01) ) / 2  - tanh( 1000*(x-0.99) ) / 2;

end

== matlab function base_lib/F0022_heatPump/F0022_vaporFraction.m ==
  data: B input; x output; B_liq input; B_vap input
function x = F0022_vaporFraction(B, B_liq, B_vap)

% B is an arbitrary thermodynamic property, ie
% specific volume, enthalpy, etc.

x = (B - B_liq) ./ (B_vap - B_liq);

end

== matlab function base_lib/F0003_pukrushpan2004/F0003_waterContent.m ==
  data: a input; lambda output
function lambda = F0003_waterContent(a)
lambda = zeros(length(a),1);
% lambda( a <= 1) = 0.043 + 17.81.*a - 39.85.*a.^2 + 36.*a.^3;
% lambda( a > 1)  = 14 + 1.4*(a-1);

lambda = 0.043 + 17.81.*a - 39.85.*a.^2 + 36.*a.^3;

end

== matlab function base_lib/F0010_gasFlow/F0010_vaporSaturationPressure.m ==
  data: T input; p_sat output
function p_sat = F0010_vaporSaturationPressure(T)
% Journal of Physical and Chemical Reference Data 31,
% 387 (2002); https://doi.org/10.1063/1.1461829
c1 =  -7.85951783;
c2 =   1.84408259;
c3 = -11.7866497;
c4 =  22.6807411;
c5 = -15.9618719;
c6 =   1.80122502;

% critical temperature & pressure
Tcrit = 647.096;
pcrit = 22.06e6;

% saturation pressure as function of temperature
p_sat = pcrit*exp(Tcrit./T .* ( ...
    c1*(1-T./Tcrit) + ...
    c2*(1-T./Tcrit).^1.5 + ...
    c3*(1-T./Tcrit).^3 + ...
    c4*(1-T./Tcrit).^3.5 + ...
    c5*(1-T./Tcrit).^4 + ...
    c6*(1-T./Tcrit).^7.5 ));

% p_sat = real(p_sat);
end

== matlab function base_lib/F0017_channelCooling/F0017_velocity.m ==
  data: W input; v output; rho input; par parameter
function v = F0017_velocity(W, rho, par)

% parameters
d   = par.d;

% area
A = pi .* d.^2 / 4;

% velocity
v = W ./ (rho .* A);

== matlab function base_lib/F0004_fluidProperties/F0004_vaporSaturationConcentration.m ==
  data: p_sat input; c_sat output; T input; par parameter
function c_sat = F0004_vaporSaturationConcentration(p_sat, T, par)
% saturation concentration
c_sat = p_sat ./ (par.R .* T);

end

== matlab function base_lib/F0025_spalFans/F0025_pressureVA164A.m ==
  data: q input; dp output; n input
function dp = F0025_pressureVA164A(q, n)

% parameters
a = [1.013138031041656e+03; -4.046095247275258e+02];

% function
dp2 = a(1) + a(2) .* q;

% affinity law
dp = dp2 .* (n./3000).^2;

end

== matlab function base_lib/F0025_spalFans/F0025_pressureVA195.m ==
  data: q input; dp output; n input
function dp = F0025_pressureVA195(q, n)

% parameters
a = [2.142485036049257e+02; -1.348961865573845e+03];

% function
dp2 = a(1) + a(2) .* q;

% affinity law
dp = dp2 .* (n./5000).^2;

end

== matlab function base_lib/F0026_turbine/F0026_turbine.m ==
  data: W input; P output; p3 input; p4 input; T3 input; N input; eta output; T4 output; par parameter
function [P, eta, T4] = F0026_turbine(W, p3, p4, T3, N, par)
D = par.D;
% x = par.x;
y = par.y;

% pressure ratio
Pi = p4./p3;

% ratio of specific heats
g = 1.4;

% efficiency
BSR = pi .* D .* N  ./ ( 60 .* sqrt(2 .* 1e3 .* T3 .* ( 1 - Pi.^((g-1)./g) ) ) );
A   = [ones(length(BSR), 1), N./sqrt(T3), (N./sqrt(T3)).^2];
B   = [A, A .* BSR, A.*BSR.^2];
eta = B * y;

% eta saturation
eta = min(eta,   1);
eta = max(eta,   0);

% Power
cp = 1e3;
P  = W .* cp .* eta .* T3 .* (1 - Pi.^((g-1)./g) );

% Temperature
T4 = T3 .* ( 1 - eta .* (1 - Pi.^((g-1)./g) ));

end

== matlab function base_lib/F0027_humidgas/F0027_hydrogenProperties.m ==
  data: p_H2 input; cp output; T input; mu output; lam output
function [cp, mu, lam] = hydrogen_properties(p_H2, T)

% parameters
Tc   = 33.145;
rhoc = 31.262;
sig  = 0.297;
ek   = 30.41;
M    = 2.01588;

% partial density
R   = 8.314;
rho = 2.016e-3 .* p_H2 ./ (R .* T);

% ideal gas heat capacity
u  = [1.616 -0.4117 -0.792 0.758 1.217]';
v  = [531 751 1989 2484 6859]';
cp = 1./(2.01568e-3) .* R .* ( 2.5 + ... 
    sum( u .* (v./T).^2 .* exp(v ./ T) ./ ( exp(v./T) - 1).^2 ));

% zero density limit viscosity
a   = [2.09630e-1, -4.55274e-1, 1.43602e-1, -3.35325e-2, 2.76981e-3];
S   = exp( sum( a .* log(T ./ ek).^(0:4), 2) );
mu0 = 0.021357 .* (M .* T).^0.5 ./ ( sig.^2 .* S );

% excess contribution density coefficient
NA  = 6.02214129e23;
b   = [-0.1870, 2.4871, 3.7151, -11.0972, 9.0965, -3.8292, 0.5166];
B   = NA .* (sig .* 1e-9).^3 .* sum( b .* (T./ek).^(0:-1:-6), 2);
mu1 = B .* mu0 ./ (M .* 1e-3);

% excess contribution intercept
Tr    = T ./ Tc;
rhor  = rho./ 90.909090909; 
c     = [6.43449673, 4.56334068e-2, 2.32797868e-1, 9.58326120e-1, 1.27941189e-1, 3.63576595e-1];
dmuh  = c(1) .* rhor.^2 .* exp( c(2) .* Tr + ...
    c(3)./Tr + ...
    c(4) .* rhor.^2 ./ (c(5) + Tr) + c(6) .* rhor.^6 );

% viscosity
mu = 1e-6 .* (mu0 + mu1 .* rho + dmuh);

% zero density limit
A1   = [-3.40976e-1,  4.58820e0, -1.45080e0, 3.26394e-1, 3.16939e-3, 1.90592e-4, -1.13900e-6];
A2   = [  1.38497e2, -2.21878e1,   4.57151e0, 1.00e0 ];
lam0 = sum(A1 .* (T./Tc).^(0:6), 2) ./ sum( A2 .* (T./Tc).^(0:3), 2);

% excess contribution
B1 = [ 3.63081e-2, -2.07629e-2, 3.14819e-2, -1.43097e-2, 1.74980e-3 ];
B2 = [ 1.83370e-3, -8.86716e-3, 1.58260e-2, -1.06283e-2, 2.80673e-3 ];
dlam = sum( (B1 + B2 .* (T./Tc) ) .* (rho./rhoc).^(1:5) , 2);

% thermal conductivity;
lam = lam0 + dlam;

end

== matlab function base_lib/F0027_humidgas/F0027_mixtureProperties.m ==
  data: cp input; cp_m output; mu input; lam input; p input; T input; mu_m output; lam_m output
function [cp_m, mu_m, lam_m] = mixture_properties(cp, mu, lam, p, T)

% molar fractions
x = p ./ sum(p,1);

% molar weights
M = [2.016e-3; 31.999e-3; 18.015e-3; 28.014e-3];

% mass fractions
M_avg = sum(x .* M);
w     = x .* M ./ M_avg;

% mixture specific heat capacity
cp_m = sum(w .* cp);

% Wilke's rule for mixture viscosity
phi  = (1 + (mu ./ mu').^0.5 .* (M' ./ M).^0.25).^2 ./ ...
    ( (4/sqrt(2)) .* (1 + (M ./ M')).^0.5 ) ;

% Eq. 13
num           = mu;
phi0          = phi;
phi0(1:5:end) = 0; 
den  = 1 + 1./x .* sum( x' .* phi0, 2);
mu_m = sum(num ./ den, 1);


% Sutherland constant
S   = [79; 90.2.*1.5; 373.15*1.5; 77.*1.5];
Sij = sqrt(S .* S');

% parameter
A  = 0.25 .* ( 1 + ( mu ./ mu' .* (M' ./ M).^0.75 .* ...
    (1 + S./T)./(1 + S'./T) ).^0.5 ).^2 .* ...
    (1 + Sij./T)./(1 + S./T);

% Eq. 11
num   = lam;
den   = 1./x .* sum( A .* x', 2);
lam_m = sum( num./den, 1); 

end

== matlab function base_lib/F0027_humidgas/F0027_nitrogenProperties.m ==
  data: p_N2 input; cp output; T input; mu output; lam output
function [cp, mu,lam] = nitrogen_properties(p_N2, T)

% Nitrogen parameters
Tc   = 126.192;  % K
rhoc = 11.1839;  % mol / dm3
pc   = 3.3958;   % MPa
M    = 28.01348; % g / mol
ek   = 98.94;    % -
sig  = 0.3656;   % nm

% partial density
R   = 8.314;
rho = 28.01348e-3 .* p_N2 ./ (R .* T);

% ideal gas heat capacity
u  = 3364.011./T;
a  = [3.5 3.066469e-6 4.701240e-9 -3.987984e-13 1.012941]';
cp = 1./28.01348e-3 .* R .* ( ...
    a(1) + a(2) .* T + a(3) .* T.^2 + a(4) .* T.^3 + ...
    a(5) .* u.^2 .* exp(u) ./ (exp(u) - 1).^2 );

% change units on density from kg / m3 --> mol / dm3
rho = 1e-3 .* rho ./ (M * 1e-3);

% reduced temperature and density
tau =  Tc ./ T;
del = rho ./ rhoc;

% dilute gas contributoin
Ts    = T ./ ek;
b     = [0.431, -0.4623, 0.08406, 0.005341, -0.00331];
Omega = exp( sum( b .* log(Ts).^(0:4), 2) ); 
mu0   = 0.0266958 .* sqrt(M .* T) ./ (sig.^2 .* Omega );

% residual contribution
N = [10.72, 0.03989, 0.001208, -7.402, 4.620];
t = [0.1, 0.25, 3.2, 0.9, 0.3];
d = [2, 10, 12, 2, 1];
l = [0, 1, 1, 2, 3];
g = [0, 1, 1, 1, 1];
mur = sum( N .* tau.^t .* del.^d .* exp( -g .* del.^l), 2);

% viscosity
mu = 1e-6 .* ( mu0 + mur );

% dilute gas thermal conductivity
N = [1.511 2.117 -3.332];
t = [0 -1.0 -0.7];
lam0 = N(1) .* mu0 + N(2) .* tau.^t(2) + N(3) .* tau.^t(3);

% residual contribution
N = [8.862 31.11 -73.13 20.03 -0.7096 0.2672];
t = [0 0.03 0.2 0.8 0.6 1.9];
d = [1    2   3   4   8  10];
l = [0 0 1 2 2 2];
g = [0 0 1 1 1 1];
lamr = sum( N .* tau.^t .* del.^d .* exp( -g .* del.^l ), 2);

% thermal conductivity
lam = 1e-3 .* ( lam0 + lamr );

end

== matlab function base_lib/F0027_humidgas/F0027_oxygenProperties.m ==
  data: p_O2 input; cp output; T input; mu output; lam output
function [cp, mu, lam] = oxygen_properties(p_O2, T)

% Oxygen parameters
Tc   = 154.581;  % K
rhoc = 13.63;  % mol / dm3
M    = 31.9988; % g / mol
ek   = 118.5;    % -
sig  = 0.3428;   % nm

% partial density
R   = 8.314;
rho = 31.9988e-3 .* p_O2 ./ (R .* T);

% ideal gas heat capacity
N   = [1.06778 3.50042 0.166961e-7 1.01258 0.944365 2242.45 11580.4];
eta = N(7) ./ T;
u   = N(6) ./ T;
cp  = 1./(31.9988e-3) .* R .* ( ...
    N(1) .* T^-1.5 + ...
    N(2) + ...
    N(3) .* T.^2 + ...
    N(4) .* u.^2 .* exp(u)./(exp(u) - 1).^2 + ...
    N(5) .* 2/3 .* eta.^2 .* exp(-eta) ./ (1 + 2/3 .* exp(-eta) ).^2 ...
    );

% change units on density from kg / m3 --> mol / dm3
rho = 1e-3 .* rho ./ (M * 1e-3);

% reduced temperature and density
tau =  Tc ./ T;
del = rho ./ rhoc;

% dilute gas contributoin
Ts    = T ./ ek;
b     = [0.431, -0.4623, 0.08406, 0.005341, -0.00331];
Omega = exp( sum( b .* log(Ts).^(0:4), 2) );
mu0   = 0.0266958 .* sqrt(M .* T) ./ (sig.^2 .* Omega );

% residual contribution
N = [17.67, 0.4042, 0.0001077, 0.3510, -13.67];
t = [0.05 0.0 2.10 0.0 0.5];
d = [1 5 12 8 1];
l = [0 0 0 1 2];
g = [0 0 0 1 1];
mur = sum( N .* tau.^t .* del.^d .* exp( -g .* del.^l), 2);

% viscosity
mu = 1e-6 .* ( mu0 + mur );

% dilute gas thermal conductivity
N = [1.036 6.283 -4.262];
t = [0 -0.9 -0.6];
lam0 = N(1) .* mu0 + N(2) .* tau.^t(2) + N(3) .* tau.^t(3);

% residual contribution
N = [15.31 8.898 -0.7336 6.728 -4.374 -0.4747];
t = [0.0 0.0 0.3 4.3 0.5 1.8];
d = [1 3 4 5 7 10];
l = [0 0 0 2 2 2];
g = [0 0 0 1 1 1];
lamr = sum( N .* tau.^t .* del.^d .* exp( -g .* del.^l ), 2);

% thermal conductivity
lam = 1e-3 .* ( lam0 + lamr );

end
